simulink model "verify_THBCreator_mdl"  (R2013b)
settings: Solver=VariableStepDiscrete  StartTime=0.0  StopTime=10.0  MaxStep=0.1  RelTol=1e-3
libraries: carnot x1
settings Model: Creator=drhf  LastModifiedBy=drhf
settings OptimizationCC: ExpressionDepthLimit=2147483647
settings DebuggingCC: StateNameClashWarn=warning
settings GRTTargetCC: CombineOutputUpdateFcns=off  GRTInterface=on

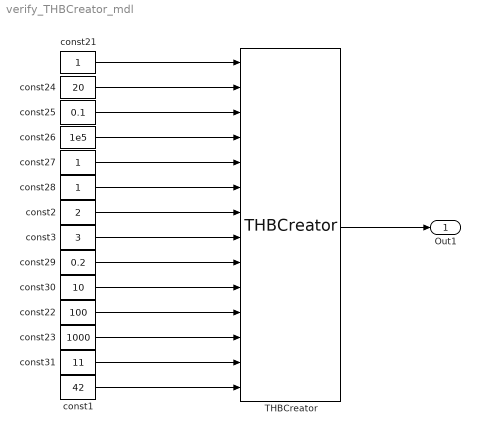
== system verify_THBCreator_mdl ==
  THBCreator : carnot/Basic/Hydraulics/THBCreator  Inport_ID=on  Inport_T=on  Inport_mdot=on  Inport_p=on  Inport_type=on  Inport_mix=on  Inport_mix2=on  Inport_mix3=on  Inport_d=on  Inport_c=on  Inport_l=on  Inport_q=on  Inport_LH=on  Inport_H=on  ID=20001  T=20  mdot=0  p=1e5  FluidType=1  FluidMix=0  FluidMix2=0  FluidMix3=0  d=0.02  c=0  l=0  q=0  LH=0  H=0  Annotation_ID=off  Annotation_T=off  Annotation_mdot=off  Annotation_p=off  Annotation_type=off  Annotation_mix=off  Annotation_mix2=off  Annotation_mix3=off  Annotation_d=off  Annotation_c=off  Annotation_l=off  Annotation_q=off  Annotation_LH=off  Annotation_H=off
  const1 : Constant  Value=42
  const2 : Constant  Value=2
  const21 : Constant
  const22 : Constant  Value=100
  const23 : Constant  Value=1000
  const24 : Constant  Value=20
  const25 : Constant  Value=0.1
  const26 : Constant  Value=1e5
  const27 : Constant
  const28 : Constant
  const29 : Constant  Value=0.2
  const3 : Constant  Value=3
  const30 : Constant  Value=10
  const31 : Constant  Value=11
  Out1 : Outport
  wires:
  THBCreator/1 -> Out1/1
  const3/1 -> THBCreator/8
  const25/1 -> THBCreator/3
  const26/1 -> THBCreator/4
  const1/1 -> THBCreator/14
  const21/1 -> THBCreator/1
  const27/1 -> THBCreator/5
  const31/1 -> THBCreator/13
  const28/1 -> THBCreator/6
  const2/1 -> THBCreator/7
  const29/1 -> THBCreator/9
  const22/1 -> THBCreator/11
  const30/1 -> THBCreator/10
  const23/1 -> THBCreator/12
  const24/1 -> THBCreator/2
